simulink model "sim_1_mixing"  (R2021a)
settings: Solver=VariableStepAuto  StartTime=0.0  StopTime=120  RelTol=1e-3
libraries: dspsrcs4 x2, commanapbnd3 x1, dspspect3 x1
settings Model: Creator=vpixx  LastModifiedBy=vpixx

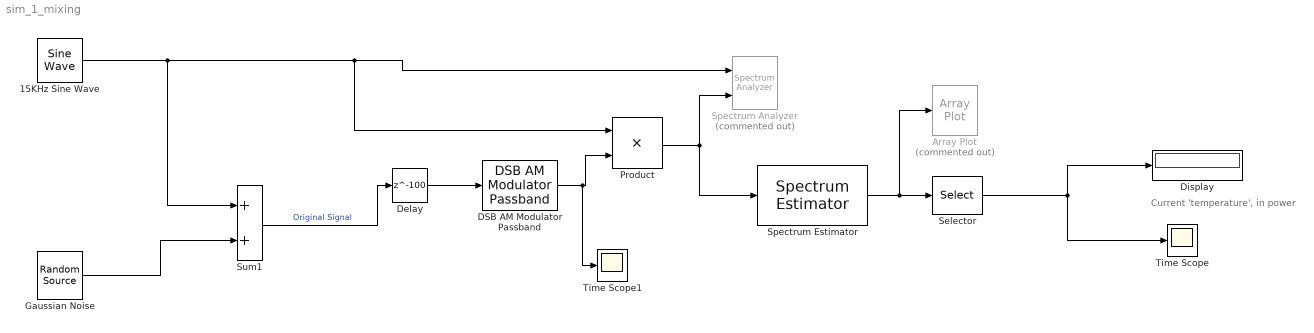
== system sim_1_mixing ==
  note: Current 'temperature', in power
  15KHz Sine Wave : dspsrcs4/Sine Wave  Amplitude=1  Frequency=15000  Phase=0  SampleMode=Discrete  OutComplex=Real  CompMethod=Trigonometric fcn  TableSize=Speed  SampleTime=1/44100  SamplesPerFrame=1  ResetState=Restart at time zero  OutputFrames=off  dataType=double  wordLen=16  udDataType=sfix(16)  fracBitsMode=Best precision  numFracBits=15  OutDataTypeStr=double  LastOutDataTypeStr=double
  Array Plot : ArrayPlot  Commented=on  WindowPosition=[-1548.000000,1151.000000,800.000000,500.000000,]  YLimits=[-35.83093547125317,14.65971224812893]  DefaultConfigurationName=dsp.scopes.ArrayPlotBlockSpecification
  DSB AM Modulator Passband : commanapbnd3/DSB AM Modulator Passband  Fc=0.01  Ph=0  Offset=0
      settings: SourceProductBaseCode=CM
  Delay : Delay  DelayLength=100  InitialCondition=0
  Display : Display
  Gaussian Noise : dspsrcs4/Random Source  SrcType=Gaussian  NormMethod=Ziggurat  CltLength=12  MinVal=0  MaxVal=1  MeanVal=0  VarVal=.20  RepMode=Specify seed  rawSeed=1234567  IsInherit=off  SampMode=Discrete  SampTime=1/44100  SampFrame=1  DataType=Double  OutComplex=Real  OutputFrames=off
  Product : Product
  Selector : Selector  NumberOfDimensions=2  InputPortWidth=3  IndexOptions=Index vector (dialog),Index vector (dialog)  Indices=1,1  OutputSizes=1,1
  Spectrum Analyzer : SpectrumAnalyzer  Commented=on  NumInputPorts=2
  Spectrum Estimator : dspspect3/Spectrum Estimator  Method=Filter bank  NumTapsPerBand=12  SpectrumType=Power  FrequencyResolutionMethod=Auto  FilterBankResolutionMethod=Auto  RBW=5  WindowLength=1024  FrequencyBandsSource=Same as input frame size  FrequencyBands=1024  FFTLengthSource=Auto  FFTLength=1024  InheritSampleRate=on  SampleRate=44100  Window=Hann  SidelobeAttenuation=60  AveragingMethod=Exponential  SpectralAverages=1  ForgettingFactorPort=off  ForgettingFactor=0.9  Overlap=0  ReferenceLoad=1  FrequencyRange=One-sided  PowerUnits=dBm  OutputMaxHoldSpectrum=off  OutputMinHoldSpectrum=off  OutputFrequencyVector=off  OutputRBW=off  SimulateUsing=Code generation
      settings: SourceProductBaseCode=DS
  Sum1 : Sum
  Time Scope : Scope
  Time Scope1 : Scope
  wires:
  Product/1 -> Spectrum Estimator/1, Spectrum Analyzer/2
  Sum1/1 -> Delay/1  "Original Signal"
  15KHz Sine Wave/1 -> Product/1, Spectrum Analyzer/1, Sum1/1
  Spectrum Estimator/1 -> Array Plot/1, Selector/1
  Gaussian Noise/1 -> Sum1/2
  Delay/1 -> DSB AM Modulator Passband/1
  DSB AM Modulator Passband/1 -> Time Scope1/1, Product/2
  Selector/1 -> Time Scope/1, Display/1
